simulink model "power_system_v2_1"  (R2015b)
settings: Solver=VariableStepAuto  StartTime=0.0  StopTime=1000  RelTol=1e-3
values from neighbouring files (symbols this model uses):
  A = [   1  -1  0   0    0 ... (first row only)    [init_power_system_v2_1.m]    (also in test1.m = [   1  -1  0   0)
  B_prime = diag(sum(Ymat,2)') - Ymat    [init_power_system_v2_1.m]    (also in test1.m = diag(sum(Ymat')) - Ymat)
  D = diag(Y)    [init_power_system_v2_1.m]    (also in test1.m)
  flowCost = 0.001    [init_power_system_v2_1.m]    (also in test1.m)
  L = 1000    [init_power_system_v2_1.m]
  maxFlowVector = [40 40 10 40 40]'    [init_power_system_v2_1.m]    (also in test1.m = [40 40 10 40]')
  minFlowVector = -[40 40 10 40 40]'    [init_power_system_v2_1.m]    (also in test1.m = -[40 40 10 40]')
  sample_time_frr_a = 10    [init_power_system_v2_1.m]
  Ymat = [0       Y_12    Y_13    0       0 ... (first row only)    [init_power_system_v2_1.m]    (also in test1.m = [   0       T_12    T_13    T_14; tieline.m = [   0       T_12    T_13    T_14)
undefined symbols (not defined in the file or in its folder): C_down, C_up, Q_max_down, Q_max_up, Q_min_down, Q_min_up
undefined symbols (not defined in the file): area_param_1, area_param_2, area_param_3, area_param_4, area_param_5
libraries: aerolibanimutils x1
settings Model: Creator=tarje  LastModifiedBy=tarje

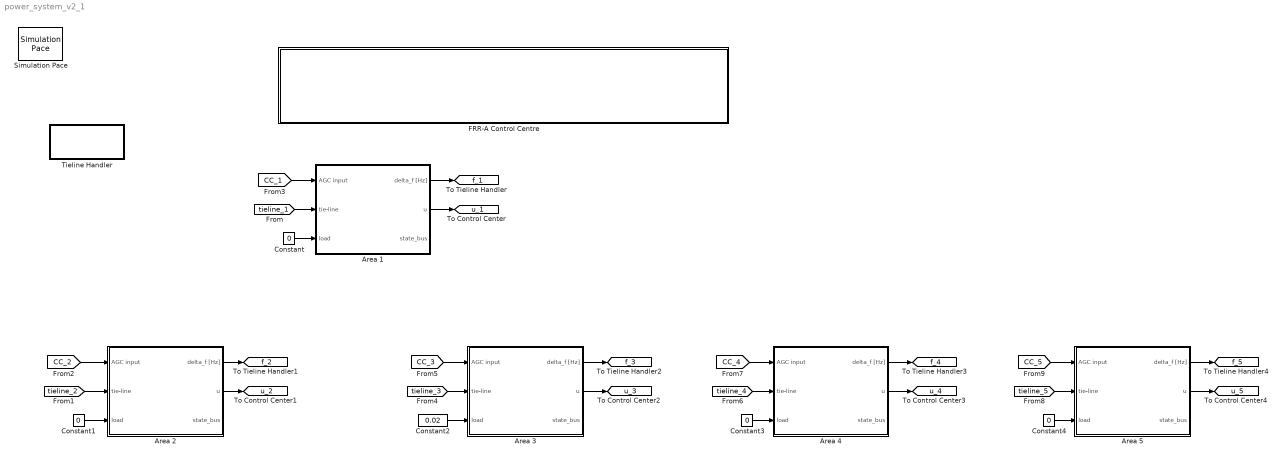
== system power_system_v2_1 ==
  Area 1 : Subsystem  mask(Power system w/ primary control){param=area_param_1}
      mask prompts: param "Area parameters"
      mask help:
      | Linear model of generator, turbine and governor with primary control. Demand estimated from secondary control loop, using ACE signal. All values are per unit delta values from a normal operating point.
      |
      | Parameters = [T_g T_t H D R]
      mask Display: % image('hydropower.jpg')
  Area 2 : Subsystem  mask(Power system w/ primary control){param=area_param_2}
      mask prompts: param "Area parameters"
      mask help:
      | Linear model of generator, turbine and governor with primary control. Demand estimated from secondary control loop, using ACE signal. All values are per unit delta values from a normal operating point.
      |
      | Parameters = [T_g T_t H D R]
      mask Display: % image('hydropower.jpg')
  Area 3 : Subsystem  mask(Power system w/ primary control){param=area_param_3}
      mask prompts: param "Area parameters"
      mask help:
      | Linear model of generator, turbine and governor with primary control. Demand estimated from secondary control loop, using ACE signal. All values are per unit delta values from a normal operating point.
      |
      | Parameters = [T_g T_t H D R]
      mask Display: % image('hydropower.jpg')
  Area 4 : Subsystem  mask(Power system w/ primary control){param=area_param_4}
      mask prompts: param "Area parameters"
      mask help:
      | Linear model of generator, turbine and governor with primary control. Demand estimated from secondary control loop, using ACE signal. All values are per unit delta values from a normal operating point.
      |
      | Parameters = [T_g T_t H D R]
      mask Display: % image('hydropower.jpg')
  Area 5 : Subsystem  mask(Power system w/ primary control){param=area_param_5}
      mask prompts: param "Area parameters"
      mask help:
      | Linear model of generator, turbine and governor with primary control. Demand estimated from secondary control loop, using ACE signal. All values are per unit delta values from a normal operating point.
      |
      | Parameters = [T_g T_t H D R]
      mask Display: % image('hydropower.jpg')
  Constant{,1,3..4} (4 alike) : Constant  Value=0
  Constant2 : Constant  Value=0.02
  "FRR-A Control Centre " : Subsystem
  Simulation Pace : aerolibanimutils/Simulation Pace  SimulationPace=1  SleepMode=MATLAB Thread  OutputPaceError=off  SampleTime=1/30
      settings: AttributesFormatString=%<SimulationPace> sec/sec
  Tieline Handler : Subsystem
  tag scope: f_1=global, f_2=global, f_3=global, f_4=global, f_5=global, u_1=global, u_2=global, u_3=global, u_4=global, u_5=global
  wires:
  [tieline_1] -> Area 1/2(tie-line)
  Constant/1 -> Area 1/3(load)
  [CC_1] -> Area 1/1(AGC input)
  Area 1/1(delta_f [Hz]) -> [f_1]
  Area 1/2(u) -> [u_1]
  [tieline_2] -> Area 2/2(tie-line)
  Constant1/1 -> Area 2/3(load)
  [CC_2] -> Area 2/1(AGC input)
  Area 2/1(delta_f [Hz]) -> [f_2]
  Area 2/2(u) -> [u_2]
  [tieline_3] -> Area 3/2(tie-line)
  Constant2/1 -> Area 3/3(load)
  [CC_3] -> Area 3/1(AGC input)
  Area 3/1(delta_f [Hz]) -> [f_3]
  Area 3/2(u) -> [u_3]
  [tieline_4] -> Area 4/2(tie-line)
  Constant3/1 -> Area 4/3(load)
  [CC_4] -> Area 4/1(AGC input)
  Area 4/1(delta_f [Hz]) -> [f_4]
  Area 4/2(u) -> [u_4]
  [tieline_5] -> Area 5/2(tie-line)
  Constant4/1 -> Area 5/3(load)
  [CC_5] -> Area 5/1(AGC input)
  Area 5/1(delta_f [Hz]) -> [f_5]
  Area 5/2(u) -> [u_5]

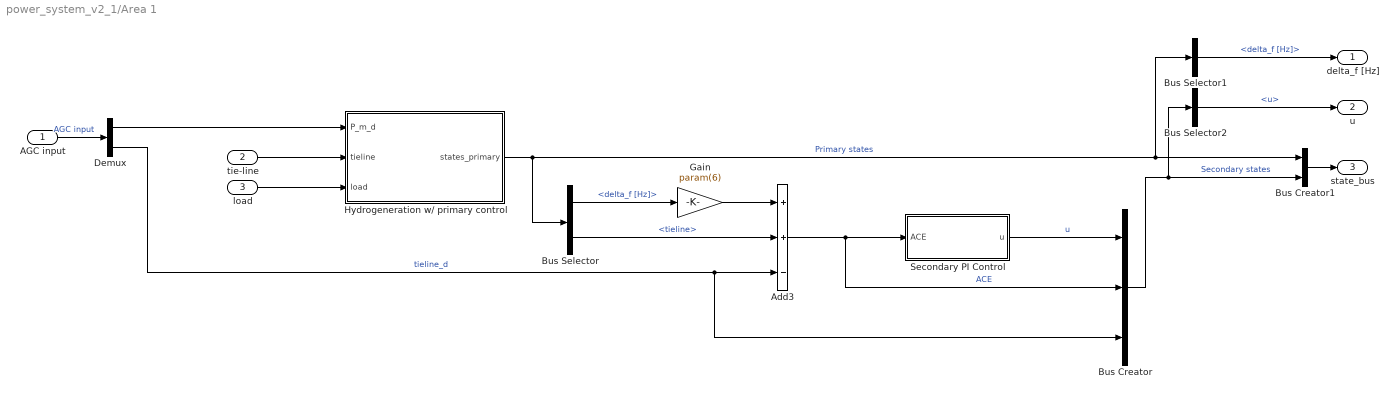
== system power_system_v2_1/Area 1 ==
  AGC input : Inport
  tie-line : Inport  Port=2
  load : Inport  Port=3
  Add3 : Sum  Inputs=++-
  Bus Creator : BusCreator  Inputs=3
  Bus Creator1 : BusCreator  Inputs=2
  Bus Selector : BusSelector  OutputSignals=delta_f [Hz],tieline
  Bus Selector1 : BusSelector  OutputSignals=delta_f [Hz]
  Bus Selector2 : BusSelector  OutputSignals=u
  Demux : Demux  Outputs=2
  Gain : Gain  Gain=param(6)
  Hydrogeneration w/ primary control : Subsystem
  Secondary PI Control : Subsystem  SystemSampleTime=sample_time_frr_a  mask(Secondary PI control){Kp=param(7), Ki=param(8)}
      mask help: Uses ace to estimate a demand for area. Gains should be negative.
  delta_f [Hz] : Outport
  u : Outport  Port=2
  state_bus : Outport  Port=3
  wires:
  Add3/1 -> Bus Creator/2, Secondary PI Control/1(ACE)  "ACE"
  Demux/2 -> Bus Creator/3, Add3/3  "tieline_d"
  AGC input/1 -> Demux/1  "AGC input"
  Demux/1 -> Hydrogeneration w/ primary control/1(P_m_d)
  tie-line/1 -> Hydrogeneration w/ primary control/2(tieline)
  load/1 -> Hydrogeneration w/ primary control/3(load)
  Hydrogeneration w/ primary control/1(states_primary) -> Bus Selector1/1, Bus Creator1/1, Bus Selector/1  "Primary states"
  Bus Selector/1 -> Gain/1  "<delta_f [Hz]>"
  Bus Selector/2 -> Add3/2  "<tieline>"
  Gain/1 -> Add3/1
  Secondary PI Control/1(u) -> Bus Creator/1  "u"
  Bus Creator/1 -> Bus Selector2/1, Bus Creator1/2  "Secondary states"
  Bus Creator1/1 -> state_bus/1
  Bus Selector1/1 -> delta_f [Hz]/1  "<delta_f [Hz]>"
  Bus Selector2/1 -> u/1  "<u>"

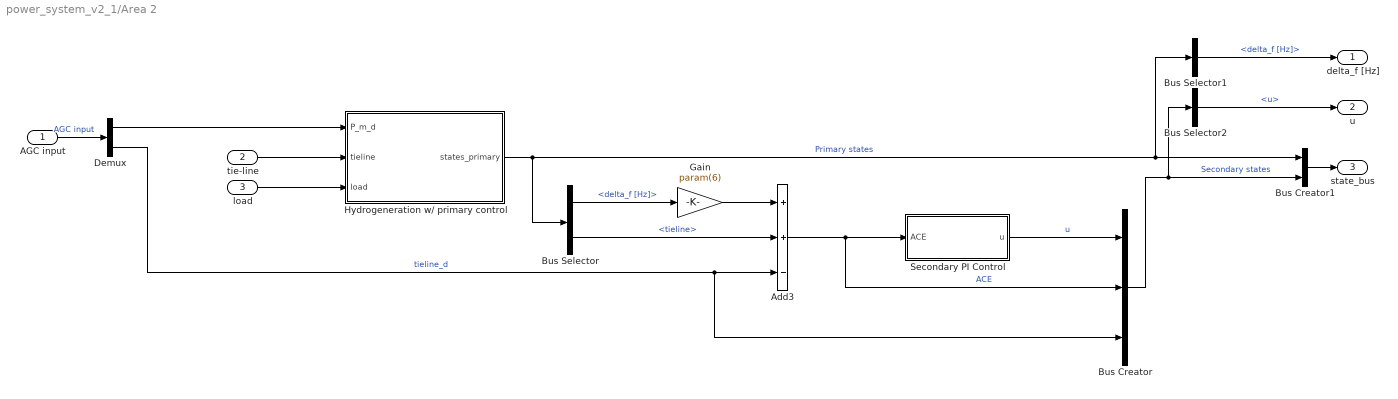
== system power_system_v2_1/Area 2 ==
  AGC input : Inport
  tie-line : Inport  Port=2
  load : Inport  Port=3
  Add3 : Sum  Inputs=++-
  Bus Creator : BusCreator  Inputs=3
  Bus Creator1 : BusCreator  Inputs=2
  Bus Selector : BusSelector  OutputSignals=delta_f [Hz],tieline
  Bus Selector1 : BusSelector  OutputSignals=delta_f [Hz]
  Bus Selector2 : BusSelector  OutputSignals=u
  Demux : Demux  Outputs=2
  Gain : Gain  Gain=param(6)
  Hydrogeneration w/ primary control : Subsystem
  Secondary PI Control : Subsystem  SystemSampleTime=sample_time_frr_a  mask(Secondary PI control){Kp=param(7), Ki=param(8)}
      mask help: Uses ace to estimate a demand for area. Gains should be negative.
  delta_f [Hz] : Outport
  u : Outport  Port=2
  state_bus : Outport  Port=3
  wires:
  Add3/1 -> Bus Creator/2, Secondary PI Control/1(ACE)  "ACE"
  Demux/2 -> Bus Creator/3, Add3/3  "tieline_d"
  AGC input/1 -> Demux/1  "AGC input"
  Demux/1 -> Hydrogeneration w/ primary control/1(P_m_d)
  tie-line/1 -> Hydrogeneration w/ primary control/2(tieline)
  load/1 -> Hydrogeneration w/ primary control/3(load)
  Hydrogeneration w/ primary control/1(states_primary) -> Bus Selector1/1, Bus Creator1/1, Bus Selector/1  "Primary states"
  Bus Selector/1 -> Gain/1  "<delta_f [Hz]>"
  Bus Selector/2 -> Add3/2  "<tieline>"
  Gain/1 -> Add3/1
  Secondary PI Control/1(u) -> Bus Creator/1  "u"
  Bus Creator/1 -> Bus Selector2/1, Bus Creator1/2  "Secondary states"
  Bus Creator1/1 -> state_bus/1
  Bus Selector1/1 -> delta_f [Hz]/1  "<delta_f [Hz]>"
  Bus Selector2/1 -> u/1  "<u>"

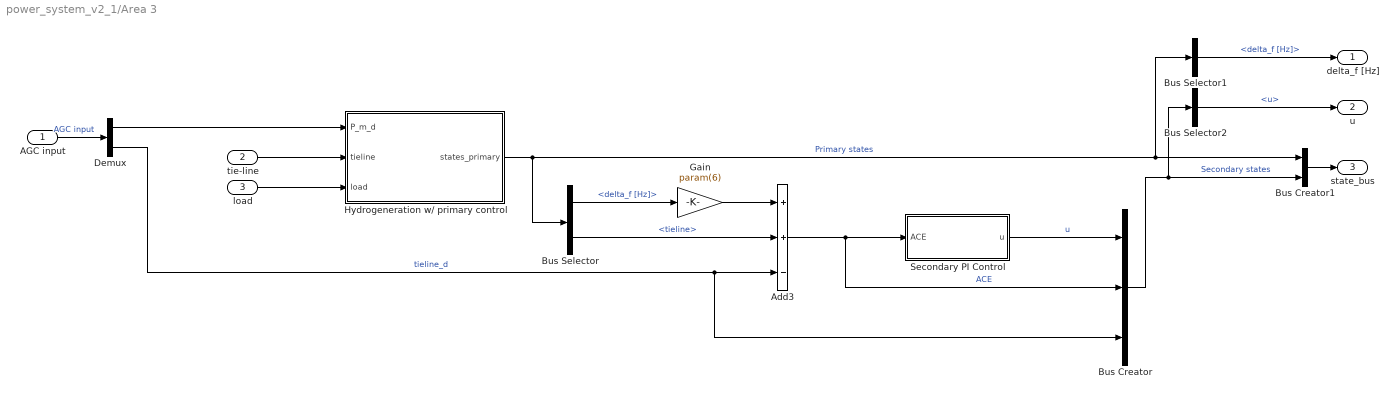
== system power_system_v2_1/Area 3 ==
  AGC input : Inport
  tie-line : Inport  Port=2
  load : Inport  Port=3
  Add3 : Sum  Inputs=++-
  Bus Creator : BusCreator  Inputs=3
  Bus Creator1 : BusCreator  Inputs=2
  Bus Selector : BusSelector  OutputSignals=delta_f [Hz],tieline
  Bus Selector1 : BusSelector  OutputSignals=delta_f [Hz]
  Bus Selector2 : BusSelector  OutputSignals=u
  Demux : Demux  Outputs=2
  Gain : Gain  Gain=param(6)
  Hydrogeneration w/ primary control : Subsystem
  Secondary PI Control : Subsystem  SystemSampleTime=sample_time_frr_a  mask(Secondary PI control){Kp=param(7), Ki=param(8)}
      mask help: Uses ace to estimate a demand for area. Gains should be negative.
  delta_f [Hz] : Outport
  u : Outport  Port=2
  state_bus : Outport  Port=3
  wires:
  Add3/1 -> Bus Creator/2, Secondary PI Control/1(ACE)  "ACE"
  Demux/2 -> Bus Creator/3, Add3/3  "tieline_d"
  AGC input/1 -> Demux/1  "AGC input"
  Demux/1 -> Hydrogeneration w/ primary control/1(P_m_d)
  tie-line/1 -> Hydrogeneration w/ primary control/2(tieline)
  load/1 -> Hydrogeneration w/ primary control/3(load)
  Hydrogeneration w/ primary control/1(states_primary) -> Bus Selector1/1, Bus Creator1/1, Bus Selector/1  "Primary states"
  Bus Selector/1 -> Gain/1  "<delta_f [Hz]>"
  Bus Selector/2 -> Add3/2  "<tieline>"
  Gain/1 -> Add3/1
  Secondary PI Control/1(u) -> Bus Creator/1  "u"
  Bus Creator/1 -> Bus Selector2/1, Bus Creator1/2  "Secondary states"
  Bus Creator1/1 -> state_bus/1
  Bus Selector1/1 -> delta_f [Hz]/1  "<delta_f [Hz]>"
  Bus Selector2/1 -> u/1  "<u>"

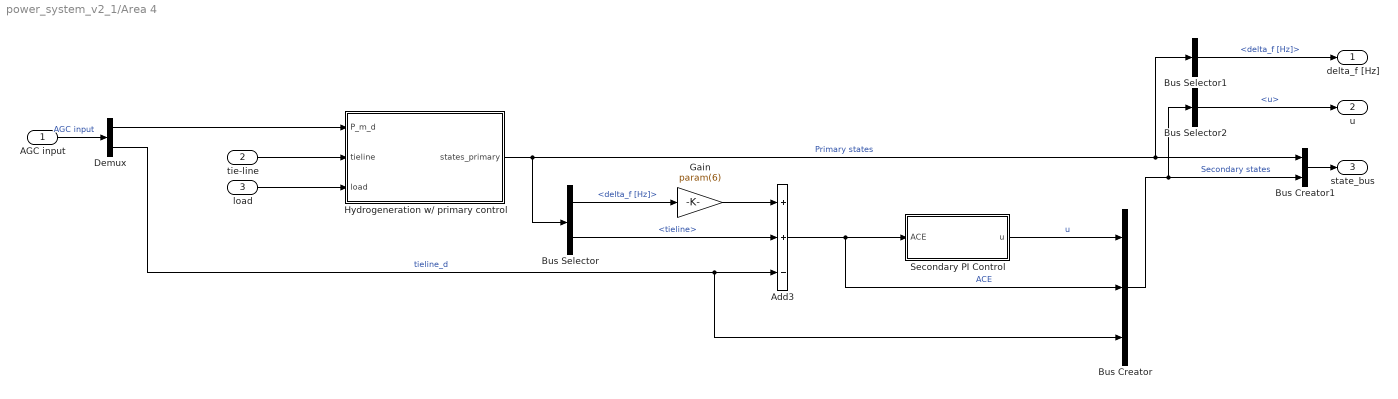
== system power_system_v2_1/Area 4 ==
  AGC input : Inport
  tie-line : Inport  Port=2
  load : Inport  Port=3
  Add3 : Sum  Inputs=++-
  Bus Creator : BusCreator  Inputs=3
  Bus Creator1 : BusCreator  Inputs=2
  Bus Selector : BusSelector  OutputSignals=delta_f [Hz],tieline
  Bus Selector1 : BusSelector  OutputSignals=delta_f [Hz]
  Bus Selector2 : BusSelector  OutputSignals=u
  Demux : Demux  Outputs=2
  Gain : Gain  Gain=param(6)
  Hydrogeneration w/ primary control : Subsystem
  Secondary PI Control : Subsystem  SystemSampleTime=sample_time_frr_a  mask(Secondary PI control){Kp=param(7), Ki=param(8)}
      mask help: Uses ace to estimate a demand for area. Gains should be negative.
  delta_f [Hz] : Outport
  u : Outport  Port=2
  state_bus : Outport  Port=3
  wires:
  Add3/1 -> Bus Creator/2, Secondary PI Control/1(ACE)  "ACE"
  Demux/2 -> Bus Creator/3, Add3/3  "tieline_d"
  AGC input/1 -> Demux/1  "AGC input"
  Demux/1 -> Hydrogeneration w/ primary control/1(P_m_d)
  tie-line/1 -> Hydrogeneration w/ primary control/2(tieline)
  load/1 -> Hydrogeneration w/ primary control/3(load)
  Hydrogeneration w/ primary control/1(states_primary) -> Bus Selector1/1, Bus Creator1/1, Bus Selector/1  "Primary states"
  Bus Selector/1 -> Gain/1  "<delta_f [Hz]>"
  Bus Selector/2 -> Add3/2  "<tieline>"
  Gain/1 -> Add3/1
  Secondary PI Control/1(u) -> Bus Creator/1  "u"
  Bus Creator/1 -> Bus Selector2/1, Bus Creator1/2  "Secondary states"
  Bus Creator1/1 -> state_bus/1
  Bus Selector1/1 -> delta_f [Hz]/1  "<delta_f [Hz]>"
  Bus Selector2/1 -> u/1  "<u>"

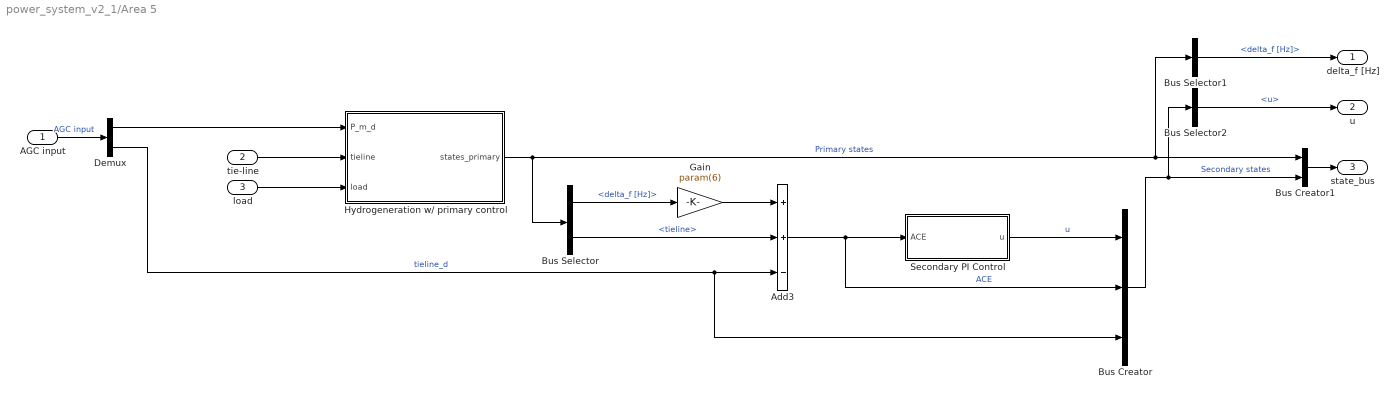
== system power_system_v2_1/Area 5 ==
  AGC input : Inport
  tie-line : Inport  Port=2
  load : Inport  Port=3
  Add3 : Sum  Inputs=++-
  Bus Creator : BusCreator  Inputs=3
  Bus Creator1 : BusCreator  Inputs=2
  Bus Selector : BusSelector  OutputSignals=delta_f [Hz],tieline
  Bus Selector1 : BusSelector  OutputSignals=delta_f [Hz]
  Bus Selector2 : BusSelector  OutputSignals=u
  Demux : Demux  Outputs=2
  Gain : Gain  Gain=param(6)
  Hydrogeneration w/ primary control : Subsystem
  Secondary PI Control : Subsystem  SystemSampleTime=sample_time_frr_a  mask(Secondary PI control){Kp=param(7), Ki=param(8)}
      mask help: Uses ace to estimate a demand for area. Gains should be negative.
  delta_f [Hz] : Outport
  u : Outport  Port=2
  state_bus : Outport  Port=3
  wires:
  Add3/1 -> Bus Creator/2, Secondary PI Control/1(ACE)  "ACE"
  Demux/2 -> Bus Creator/3, Add3/3  "tieline_d"
  AGC input/1 -> Demux/1  "AGC input"
  Demux/1 -> Hydrogeneration w/ primary control/1(P_m_d)
  tie-line/1 -> Hydrogeneration w/ primary control/2(tieline)
  load/1 -> Hydrogeneration w/ primary control/3(load)
  Hydrogeneration w/ primary control/1(states_primary) -> Bus Selector1/1, Bus Creator1/1, Bus Selector/1  "Primary states"
  Bus Selector/1 -> Gain/1  "<delta_f [Hz]>"
  Bus Selector/2 -> Add3/2  "<tieline>"
  Gain/1 -> Add3/1
  Secondary PI Control/1(u) -> Bus Creator/1  "u"
  Bus Creator/1 -> Bus Selector2/1, Bus Creator1/2  "Secondary states"
  Bus Creator1/1 -> state_bus/1
  Bus Selector1/1 -> delta_f [Hz]/1  "<delta_f [Hz]>"
  Bus Selector2/1 -> u/1  "<u>"

== system power_system_v2_1/FRR-A Control Centre  ==
  Control Signals to Areas : Subsystem
  Demux : Demux  Outputs=2
  Gain : Gain  Gain=L
  Gain1 : Gain  Gain=1/L
  Manual Switch : ManualSwitch  CurrentSetting=0
  No AGC : Subsystem  Commented=on
  Optimal FFR-A : Subsystem
  "Standard AGC, zero tieline" : Subsystem
  u from all areas : Subsystem
  wires:
  u from all areas/1(u) -> No AGC/1(u1), "Standard AGC, zero tieline"/1(u1), Gain/1
  Demux/1 -> Control Signals to Areas/1("AGC set-points ")
  Demux/2 -> Control Signals to Areas/2(tieline_d)
  "Standard AGC, zero tieline"/1(control action1) -> Manual Switch/1
  Optimal FFR-A/1(control action) -> Gain1/1
  Manual Switch/1 -> Demux/1
  Gain/1 -> Optimal FFR-A/1(u)
  Gain1/1 -> Manual Switch/2

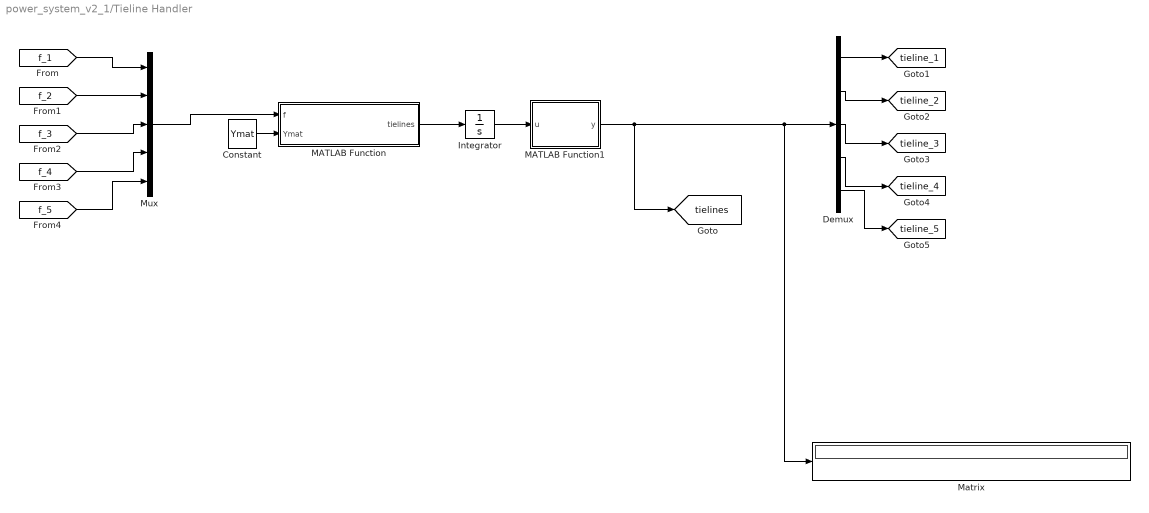
== system power_system_v2_1/Tieline Handler ==
  Constant : Constant  Value=Ymat
  Demux : Demux  Outputs=5
  Integrator : Integrator
  MATLAB Function : MATLAB Function  TreatAsAtomicUnit=on
  MATLAB Function1 : MATLAB Function  TreatAsAtomicUnit=on
  Matrix : Display
  Mux : Mux  Inputs=5
  tag scope: tieline_1=global, tieline_2=global, tieline_3=global, tieline_4=global, tieline_5=global, tielines=global
  wires:
  [f_1] -> Mux/1
  [f_2] -> Mux/2
  [f_3] -> Mux/3
  [f_4] -> Mux/4
  Mux/1 -> MATLAB Function/1(f)
  Constant/1 -> MATLAB Function/2(Ymat)
  MATLAB Function/1(tielines) -> Integrator/1
  Integrator/1 -> MATLAB Function1/1(u)
  MATLAB Function1/1(y) -> [tielines], Matrix/1, Demux/1
  Demux/1 -> [tieline_1]
  Demux/3 -> [tieline_3]
  Demux/4 -> [tieline_4]
  Demux/2 -> [tieline_2]
  [f_5] -> Mux/5
  Demux/5 -> [tieline_5]

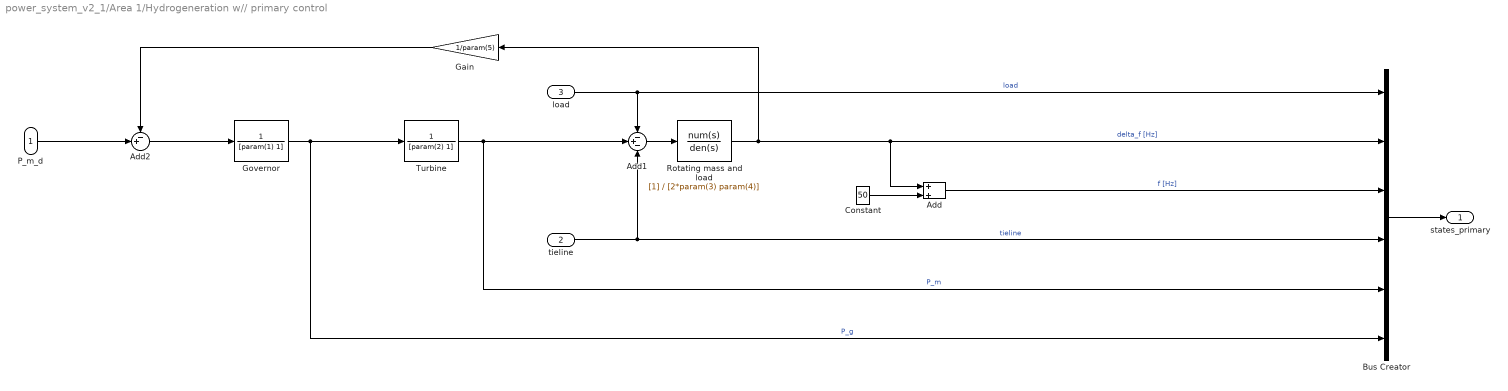
== system power_system_v2_1/Area 1/Hydrogeneration w// primary control ==
  P_m_d : Inport
  tieline : Inport  Port=2
  load : Inport  Port=3
  Add : Sum
  Add1 : Sum  Inputs=-+-
  Add2 : Sum  Inputs=-+|
  Bus Creator : BusCreator  Inputs=6
  Constant : Constant  Value=50
  Gain : Gain  Gain=1/param(5)
  Governor : TransferFcn  Denominator=[param(1) 1]
  Rotating mass and load : TransferFcn  Denominator=[2*param(3) param(4)]
  Turbine : TransferFcn  Denominator=[param(2) 1]
  states_primary : Outport
  wires:
  Gain/1 -> Add2/1
  Turbine/1 -> Bus Creator/5, Add1/2  "P_m"
  Rotating mass and load/1 -> Add/1, Bus Creator/2, Gain/1  "delta_f [Hz]"
  load/1 -> Add1/1, Bus Creator/1  "load"
  Add2/1 -> Governor/1
  Governor/1 -> Bus Creator/6, Turbine/1  "P_g"
  Add1/1 -> Rotating mass and load/1
  P_m_d/1 -> Add2/2
  tieline/1 -> Add1/3, Bus Creator/4  "tieline"
  Constant/1 -> Add/2
  Add/1 -> Bus Creator/3  "f [Hz]"
  Bus Creator/1 -> states_primary/1

== system power_system_v2_1/Area 1/Secondary PI Control ==
  ACE : Inport
  Gain : Gain  Gain=param(8)
  Integrator : Integrator
  u : Outport
  wires:
  Gain/1 -> Integrator/1
  Integrator/1 -> u/1
  ACE/1 -> Gain/1

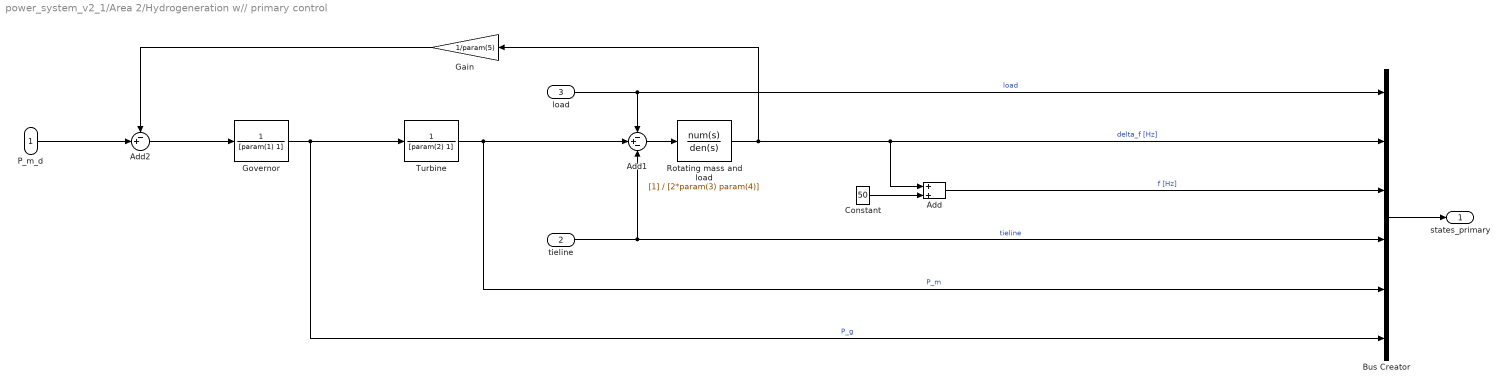
== system power_system_v2_1/Area 2/Hydrogeneration w// primary control ==
  P_m_d : Inport
  tieline : Inport  Port=2
  load : Inport  Port=3
  Add : Sum
  Add1 : Sum  Inputs=-+-
  Add2 : Sum  Inputs=-+|
  Bus Creator : BusCreator  Inputs=6
  Constant : Constant  Value=50
  Gain : Gain  Gain=1/param(5)
  Governor : TransferFcn  Denominator=[param(1) 1]
  Rotating mass and load : TransferFcn  Denominator=[2*param(3) param(4)]
  Turbine : TransferFcn  Denominator=[param(2) 1]
  states_primary : Outport
  wires:
  Gain/1 -> Add2/1
  Turbine/1 -> Bus Creator/5, Add1/2  "P_m"
  Rotating mass and load/1 -> Add/1, Bus Creator/2, Gain/1  "delta_f [Hz]"
  load/1 -> Add1/1, Bus Creator/1  "load"
  Add2/1 -> Governor/1
  Governor/1 -> Bus Creator/6, Turbine/1  "P_g"
  Add1/1 -> Rotating mass and load/1
  P_m_d/1 -> Add2/2
  tieline/1 -> Add1/3, Bus Creator/4  "tieline"
  Constant/1 -> Add/2
  Add/1 -> Bus Creator/3  "f [Hz]"
  Bus Creator/1 -> states_primary/1

== system power_system_v2_1/Area 2/Secondary PI Control ==
  ACE : Inport
  Gain : Gain  Gain=param(8)
  Integrator : Integrator
  u : Outport
  wires:
  Gain/1 -> Integrator/1
  Integrator/1 -> u/1
  ACE/1 -> Gain/1

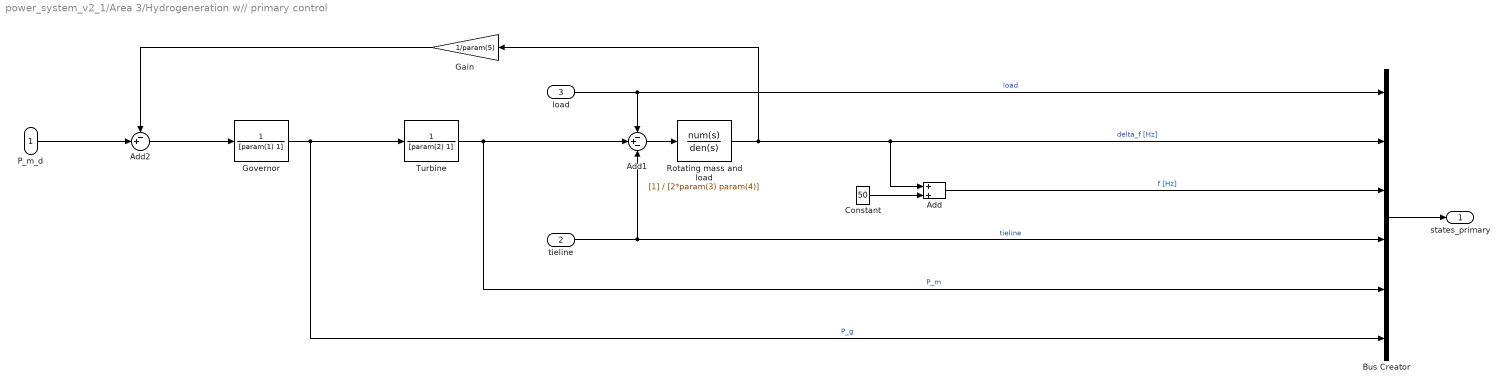
== system power_system_v2_1/Area 3/Hydrogeneration w// primary control ==
  P_m_d : Inport
  tieline : Inport  Port=2
  load : Inport  Port=3
  Add : Sum
  Add1 : Sum  Inputs=-+-
  Add2 : Sum  Inputs=-+|
  Bus Creator : BusCreator  Inputs=6
  Constant : Constant  Value=50
  Gain : Gain  Gain=1/param(5)
  Governor : TransferFcn  Denominator=[param(1) 1]
  Rotating mass and load : TransferFcn  Denominator=[2*param(3) param(4)]
  Turbine : TransferFcn  Denominator=[param(2) 1]
  states_primary : Outport
  wires:
  Gain/1 -> Add2/1
  Turbine/1 -> Bus Creator/5, Add1/2  "P_m"
  Rotating mass and load/1 -> Add/1, Bus Creator/2, Gain/1  "delta_f [Hz]"
  load/1 -> Add1/1, Bus Creator/1  "load"
  Add2/1 -> Governor/1
  Governor/1 -> Bus Creator/6, Turbine/1  "P_g"
  Add1/1 -> Rotating mass and load/1
  P_m_d/1 -> Add2/2
  tieline/1 -> Add1/3, Bus Creator/4  "tieline"
  Constant/1 -> Add/2
  Add/1 -> Bus Creator/3  "f [Hz]"
  Bus Creator/1 -> states_primary/1

== system power_system_v2_1/Area 3/Secondary PI Control ==
  ACE : Inport
  Gain : Gain  Gain=param(8)
  Integrator : Integrator
  u : Outport
  wires:
  Gain/1 -> Integrator/1
  Integrator/1 -> u/1
  ACE/1 -> Gain/1

== system power_system_v2_1/Area 4/Hydrogeneration w// primary control ==
  P_m_d : Inport
  tieline : Inport  Port=2
  load : Inport  Port=3
  Add : Sum
  Add1 : Sum  Inputs=-+-
  Add2 : Sum  Inputs=-+|
  Bus Creator : BusCreator  Inputs=6
  Constant : Constant  Value=50
  Gain : Gain  Gain=1/param(5)
  Governor : TransferFcn  Denominator=[param(1) 1]
  Rotating mass and load : TransferFcn  Denominator=[2*param(3) param(4)]
  Turbine : TransferFcn  Denominator=[param(2) 1]
  states_primary : Outport
  wires:
  Gain/1 -> Add2/1
  Turbine/1 -> Bus Creator/5, Add1/2  "P_m"
  Rotating mass and load/1 -> Add/1, Bus Creator/2, Gain/1  "delta_f [Hz]"
  load/1 -> Add1/1, Bus Creator/1  "load"
  Add2/1 -> Governor/1
  Governor/1 -> Bus Creator/6, Turbine/1  "P_g"
  Add1/1 -> Rotating mass and load/1
  P_m_d/1 -> Add2/2
  tieline/1 -> Add1/3, Bus Creator/4  "tieline"
  Constant/1 -> Add/2
  Add/1 -> Bus Creator/3  "f [Hz]"
  Bus Creator/1 -> states_primary/1

== system power_system_v2_1/Area 4/Secondary PI Control ==
  ACE : Inport
  Gain : Gain  Gain=param(8)
  Integrator : Integrator
  u : Outport
  wires:
  Gain/1 -> Integrator/1
  Integrator/1 -> u/1
  ACE/1 -> Gain/1

== system power_system_v2_1/Area 5/Hydrogeneration w// primary control ==
  P_m_d : Inport
  tieline : Inport  Port=2
  load : Inport  Port=3
  Add : Sum
  Add1 : Sum  Inputs=-+-
  Add2 : Sum  Inputs=-+|
  Bus Creator : BusCreator  Inputs=6
  Constant : Constant  Value=50
  Gain : Gain  Gain=1/param(5)
  Governor : TransferFcn  Denominator=[param(1) 1]
  Rotating mass and load : TransferFcn  Denominator=[2*param(3) param(4)]
  Turbine : TransferFcn  Denominator=[param(2) 1]
  states_primary : Outport
  wires:
  Gain/1 -> Add2/1
  Turbine/1 -> Bus Creator/5, Add1/2  "P_m"
  Rotating mass and load/1 -> Add/1, Bus Creator/2, Gain/1  "delta_f [Hz]"
  load/1 -> Add1/1, Bus Creator/1  "load"
  Add2/1 -> Governor/1
  Governor/1 -> Bus Creator/6, Turbine/1  "P_g"
  Add1/1 -> Rotating mass and load/1
  P_m_d/1 -> Add2/2
  tieline/1 -> Add1/3, Bus Creator/4  "tieline"
  Constant/1 -> Add/2
  Add/1 -> Bus Creator/3  "f [Hz]"
  Bus Creator/1 -> states_primary/1

== system power_system_v2_1/Area 5/Secondary PI Control ==
  ACE : Inport
  Gain : Gain  Gain=param(8)
  Integrator : Integrator
  u : Outport
  wires:
  Gain/1 -> Integrator/1
  Integrator/1 -> u/1
  ACE/1 -> Gain/1

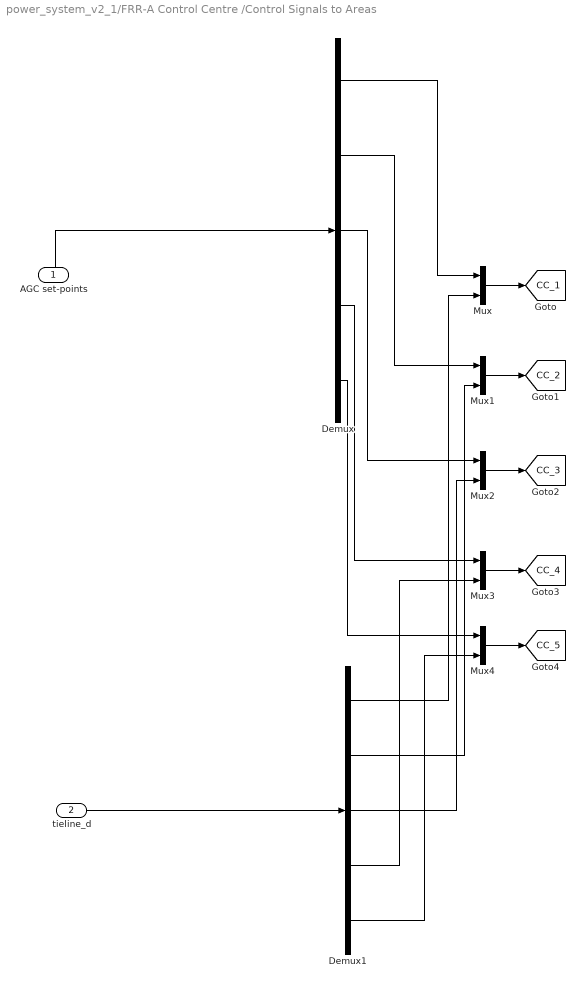
== system power_system_v2_1/FRR-A Control Centre /Control Signals to Areas ==
  "AGC set-points " : Inport
  tieline_d : Inport  Port=2
  Demux : Demux  Outputs=5
  Demux1 : Demux  Outputs=5
  Mux{,1..4} (5 alike) : Mux  Inputs=2
  tag scope: CC_1=global, CC_2=global, CC_3=global, CC_4=global, CC_5=global
  wires:
  Mux/1 -> [CC_1]
  Demux/4 -> Mux3/1
  Demux1/1 -> Mux/2
  Demux/3 -> Mux2/1
  Demux/1 -> Mux/1
  tieline_d/1 -> Demux1/1
  "AGC set-points "/1 -> Demux/1
  Mux1/1 -> [CC_2]
  Mux3/1 -> [CC_4]
  Mux2/1 -> [CC_3]
  Demux1/3 -> Mux2/2
  Demux1/2 -> Mux1/2
  Demux1/4 -> Mux3/2
  Demux/2 -> Mux1/1
  Mux4/1 -> [CC_5]
  Demux/5 -> Mux4/1
  Demux1/5 -> Mux4/2

== system power_system_v2_1/FRR-A Control Centre /No AGC ==
  u1 : Inport
  Gain : Gain  Gain=0
  Mux1 : Mux  Inputs=2
  control action1 : Outport
  wires:
  Mux1/1 -> control action1/1
  u1/1 -> Gain/1
  Gain/1 -> Mux1/1, Mux1/2

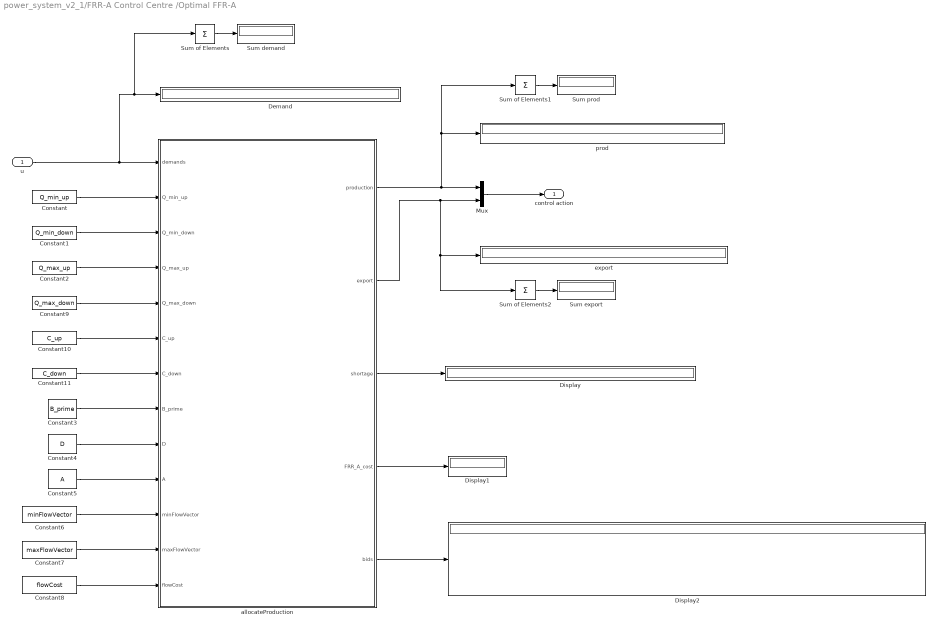
== system power_system_v2_1/FRR-A Control Centre /Optimal FFR-A ==
  u : Inport
  Constant : Constant  Value=Q_min_up
  Constant1 : Constant  Value=Q_min_down
  Constant10 : Constant  Value=C_up
  Constant11 : Constant  Value=C_down
  Constant2 : Constant  Value=Q_max_up
  Constant3 : Constant  Value=B_prime
  Constant4 : Constant  Value=D
  Constant5 : Constant  Value=A
  Constant6 : Constant  Value=minFlowVector
  Constant7 : Constant  Value=maxFlowVector
  Constant8 : Constant  Value=flowCost
  Constant9 : Constant  Value=Q_max_down
  Demand : Display
  Display : Display
  Display1 : Display
  Display2 : Display
  Mux : Mux  Inputs=2
  Sum demand : Display
  Sum export : Display
  Sum of Elements : Sum  Inputs=+
  Sum of Elements1 : Sum  Inputs=+
  Sum of Elements2 : Sum  Inputs=+
  Sum prod : Display
  allocateProduction : MATLAB Function  TreatAsAtomicUnit=on  SystemSampleTime=sample_time_frr_a
  export : Display
  prod : Display
  control action : Outport
  wires:
  Mux/1 -> control action/1
  Constant3/1 -> allocateProduction/8(B_prime)
  Constant4/1 -> allocateProduction/9(D)
  Constant5/1 -> allocateProduction/10(A)
  Constant6/1 -> allocateProduction/11(minFlowVector)
  Constant7/1 -> allocateProduction/12(maxFlowVector)
  Constant8/1 -> allocateProduction/13(flowCost)
  allocateProduction/3(shortage) -> Display/1
  allocateProduction/4(FRR_A_cost) -> Display1/1
  allocateProduction/5(bids) -> Display2/1
  Constant/1 -> allocateProduction/2(Q_min_up)
  Constant1/1 -> allocateProduction/3(Q_min_down)
  Constant2/1 -> allocateProduction/4(Q_max_up)
  Constant9/1 -> allocateProduction/5(Q_max_down)
  Constant10/1 -> allocateProduction/6(C_up)
  Constant11/1 -> allocateProduction/7(C_down)
  u/1 -> Sum of Elements/1, Demand/1, allocateProduction/1(demands)
  Sum of Elements/1 -> Sum demand/1
  allocateProduction/1(production) -> Sum of Elements1/1, prod/1, Mux/1
  Sum of Elements1/1 -> Sum prod/1
  allocateProduction/2(export) -> Sum of Elements2/1, export/1, Mux/2
  Sum of Elements2/1 -> Sum export/1

== system power_system_v2_1/FRR-A Control Centre /Standard AGC, zero tieline ==
  u1 : Inport
  Gain : Gain  Gain=0
  Mux1 : Mux  Inputs=2
  control action1 : Outport
  wires:
  Mux1/1 -> control action1/1
  u1/1 -> Gain/1, Mux1/1
  Gain/1 -> Mux1/2

== system power_system_v2_1/FRR-A Control Centre /u from all areas ==
  Mux4 : Mux  Inputs=5
  u : Outport
  wires:
  Mux4/1 -> u/1
  [u_4] -> Mux4/4
  [u_1] -> Mux4/1
  [u_2] -> Mux4/2
  [u_3] -> Mux4/3
  [u_5] -> Mux4/5

== matlab function power_system_v2_1/FRR-A Control Centre /Optimal FFR-A/allocateProduction ==
  data: demands input; production output; Q_min_up input; Q_min_down input; Q_max_up input; Q_max_down input; C_up input; C_down input; B_prime input; D input; A input; minFlowVector input; maxFlowVector input; export output; shortage output; FRR_A_cost output; flowCost input; bids output
function [production, export, shortage, FRR_A_cost, bids] = allocateProduction(demands, Q_min_up, Q_min_down, Q_max_up, Q_max_down, C_up, C_down, B_prime, D, A, minFlowVector, maxFlowVector, flowCost)
coder.extrinsic('yalmip_power_flow')

total_demand = sum(demands);

[N_up, M_up] = size(Q_max_up);
[N_down, M_down] = size(Q_max_down);
N = max(N_up, N_down);
M = max(M_up, M_down);

% Choose UP or DOWN bids
Q_min = Q_min_up;
Q_max = Q_max_up;
C = C_up;
bids_used = zeros(N_up, M_up);
if total_demand < 0
    Q_min = Q_min_down;
    Q_max = Q_max_down;
    C = C_down;
    bids_used = zeros(N_down, M_down);
end

% Declare sizes of return variables before Matlab fcn is called
production = zeros(N,1);
export = zeros(N,1);
shortage = zeros(N,1);
FRR_A_cost = 0;
bids = zeros(N, M);

[production, export, shortage, bids_used, FRR_A_cost] = yalmip_power_flow(demands, Q_min, Q_max, C, B_prime, D, A, minFlowVector, maxFlowVector, flowCost);

[n, m] = size(bids_used);
for i = 1:n
    for j = 1:m
        bids(i,j) = bids_used(i,j);
    end
end

== matlab function power_system_v2_1/Tieline Handler/MATLAB Function ==
  data: f input; tielines output; Ymat input
function tielines = matrixOperations(f, Ymat)
    
N = length(f);

% Create delta_f
f_ones = ones(N);
f_hor = zeros(N);
f_ver = zeros(N);
for i = 1:N
    f_hor(i,:) = f(i) .* f_ones(i,:); 
    f_ver(:,i) = f(i) .* f_ones(:,i);
end
delta_f = f_hor - f_ver;

% Multiply delta_f with admittance and 2PI
tielines = delta_f .* Ymat .* 2 * pi;

== matlab function power_system_v2_1/Tieline Handler/MATLAB Function1 ==
  data: u input; y output
function y = sumRows(u)
y = sum(u,2);
